simulink model "GRPsimWorkingPID"  (R2024b)
settings: Solver=FixedStepAuto  StartTime=0.0  StopTime=15  FixedStep=.0001  RelTol=1e-3
libraries: matrix_library x2, slpidlib x2, simulink x1, shared6dof x1
settings Model: Creator=aniketray  LastModifiedBy=aniketray

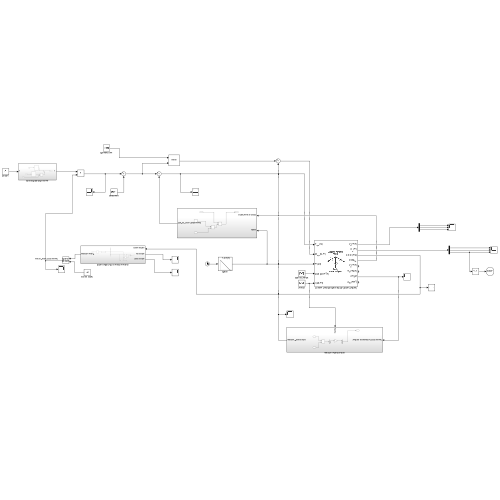
[thumbnail: Simulink's stored preview of the top-level diagram]
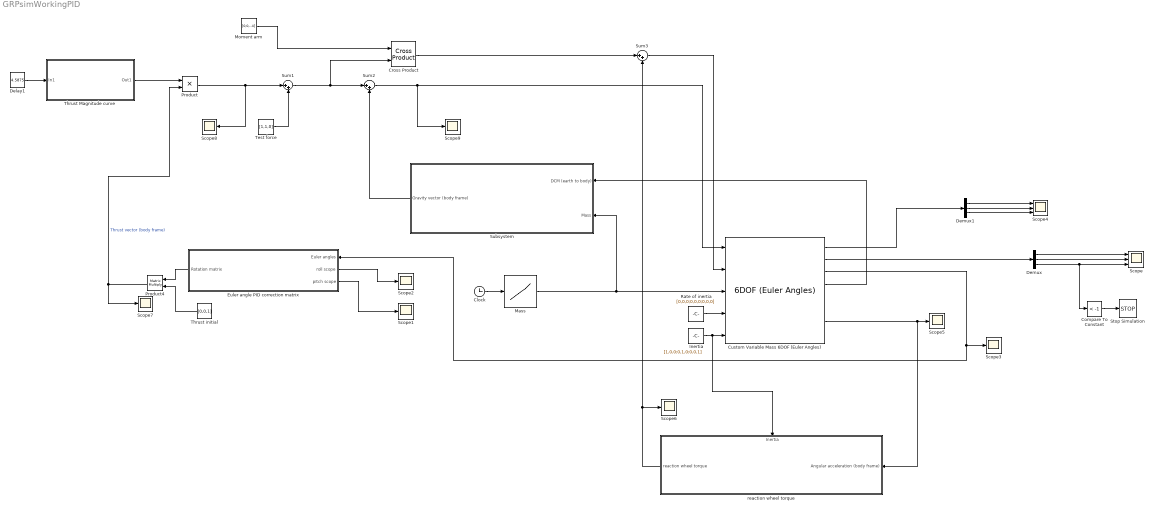
== system GRPsimWorkingPID ==
  Clock : Clock
  Compare To Constant : simulink/Logic and Bit Operations/Compare To Constant  relop=<  const=-1  OutDataTypeStr=boolean
  Cross Product : matrix_library/Cross Product
  Custom Variable Mass 6DOF (Euler Angles) : shared6dof/6DOF (Euler Angles)  units=Metric (MKS)  mtype=Custom Variable  rep=Euler Angles  xme_0=[0 0 0]  Vm_0=[0 0 0]  eul_0=[0,0,0]  pm_0=[0 0 0]  mass_0=1.0  mass_e=0.5  mass_f=2.0  inertia=eye(3)  inertia_e=eye(3)  inertia_f=2*eye(3)  k_quat=1.0  vre_flag=off  abi_flag=off  aMode=0  xme_statename=''  Vm_statename=''  eul_statename=''  quat_statename=''  pm_statename=''  mass_statename=''
      settings: LibrarySourceBlock=aerolib6dof2/Custom Variable Mass 6DOF (Euler Angles)
  Delay1 : Constant  Value=4.5875
  Demux : Demux  Outputs=3
  Demux1 : Demux  Outputs=3
  Euler angle PID correction matrix : Subsystem
      settings: PortSchema="{\"entries\":[{\"content\":{\"sides\":[{\"content\":{\"connectorIds\":[\"Out3\"]},\"type\":\"ConnectorPlacement.EquallySpacedRectSide\",\"uuid\":\"4ccd5e81-a240-4cab-acd1-338a2978d205\"},{\"content\":{\"connectorIds\":[\"In1\",\"Out1\",\"Out2\"],\"side\":\"RIGHT\"},\"type\":\"ConnectorPlacement.EquallySpacedRectSide\",\"uuid\":\"d7567d63-1202-4d9d-801d-ff17514df0c0\"},{\"content\":{\"side\":\"TOP\"},\"type\":\"ConnectorPlacement.EquallySpacedRectSide\",\"uuid\":\"5df3b33a-8f82-4d1a-a425-55f6edba809c\"}]},\"type\":\"ConnectorPlacement.EquallySpacedConnector\",\"uuid\":\"f1e1a38e-7b59-4704-87fe-778c34e8f949\"}],\"packageUris\":[\"http://schema.mathworks.com/mf0/Connector/R2020b\"],\"version\":\"1.0\"}"
  Inertia : Constant  Value=[1,0,0;0,1,0;0,0,1]
  Mass : Lookup_n-D  NumberOfTableDimensions=1  BreakpointsForDimension1=[0,3.45, 4]  Table=[1.2+0.06,1.2, 1.2]  InternalRulePriority=Speed  RndMeth=Simplest
  Moment arm : Constant  Value=[0,0,-.4]
  Product : Product
  Product4 : Product  Multiplication=Matrix(*)
  Rate of inertia : Constant  Value=[0,0,0;0,0,0;0,0,0]
  Scope : Scope  NumInputPorts=3
  Scope{1..3,5..9} (8 alike) : Scope
  Scope4 : Scope  NumInputPorts=3
  Stop Simulation : Stop
  Subsystem : Subsystem
  Sum1 : Sum  Inputs=|++
  Sum2 : Sum  Inputs=|++
  Sum3 : Sum  Inputs=|++
  Test force : Constant  Value=[1,1,0]
  Thrust Magnitude curve : Subsystem
  Thrust initial : Constant  Value=[0,0,1]
  reaction wheel torque : Subsystem
      settings: PortSchema="{\"entries\":[{\"content\":{\"sides\":[{\"content\":{\"connectorIds\":[\"In1\"]},\"type\":\"ConnectorPlacement.EquallySpacedRectSide\",\"uuid\":\"46941002-b8ec-4e8b-b9ab-4b9579ab10b5\"},{\"content\":{\"connectorIds\":[\"Out1\"],\"side\":\"RIGHT\"},\"type\":\"ConnectorPlacement.EquallySpacedRectSide\",\"uuid\":\"1b2f1bb1-3d36-42b5-8b8e-f1ef3188e1b6\"},{\"content\":{\"connectorIds\":[\"In2\"],\"side\":\"TOP\"},\"type\":\"ConnectorPlacement.EquallySpacedRectSide\",\"uuid\":\"06d0f9d8-e2f9-43b1-897a-1ea954ff583c\"}]},\"type\":\"ConnectorPlacement.EquallySpacedConnector\",\"uuid\":\"b4c30b9c-3a46-4044-8574-7f149b1eb989\"}],\"packageUris\":[\"http://schema.mathworks.com/mf0/Connector/R2020b\"],\"version\":\"1.0\"}"
  wires:
  Demux/2 -> Scope/2
  Demux/3 -> Scope/3, Compare To Constant/1
  Demux/1 -> Scope/1
  Compare To Constant/1 -> Stop Simulation/1
  Rate of inertia/1 -> Custom Variable Mass 6DOF (Euler Angles)/4
  Inertia/1 -> reaction wheel torque/2(Inertia), Custom Variable Mass 6DOF (Euler Angles)/5
  Custom Variable Mass 6DOF (Euler Angles)/2 -> Demux/1
  Clock/1 -> Mass/1
  Mass/1 -> Custom Variable Mass 6DOF (Euler Angles)/3, Subsystem/2(Mass)
  Product/1 -> Sum1/1, Scope8/1
  Sum2/1 -> Custom Variable Mass 6DOF (Euler Angles)/1, Scope9/1
  Demux1/1 -> Scope4/1
  Demux1/2 -> Scope4/2
  Demux1/3 -> Scope4/3
  Custom Variable Mass 6DOF (Euler Angles)/1 -> Demux1/1
  Moment arm/1 -> Cross Product/1
  Cross Product/1 -> Sum3/1
  Sum3/1 -> Custom Variable Mass 6DOF (Euler Angles)/2
  Custom Variable Mass 6DOF (Euler Angles)/3 -> Euler angle PID correction matrix/1(Euler angles), Scope3/1
  Thrust initial/1 -> Product4/2
  Product4/1 -> Product/2, Scope7/1  "Thrust vector (body frame)"
  Custom Variable Mass 6DOF (Euler Angles)/7 -> reaction wheel torque/1(Angular acceleration (body frame)), Scope5/1
  Delay1/1 -> Thrust Magnitude curve/1(In1)
  Thrust Magnitude curve/1(Out1) -> Product/1
  Euler angle PID correction matrix/3(Rotation matrix) -> Product4/1
  Euler angle PID correction matrix/1(roll scope) -> Scope2/1
  Euler angle PID correction matrix/2(pitch scope) -> Scope1/1
  Custom Variable Mass 6DOF (Euler Angles)/4 -> Subsystem/1(DCM (earth to body))
  Subsystem/1(Gravity vector (body frame)) -> Sum2/2
  Sum1/1 -> Cross Product/2, Sum2/1
  Test force/1 -> Sum1/2
  reaction wheel torque/1(reaction wheel torque) -> Scope6/1, Sum3/2

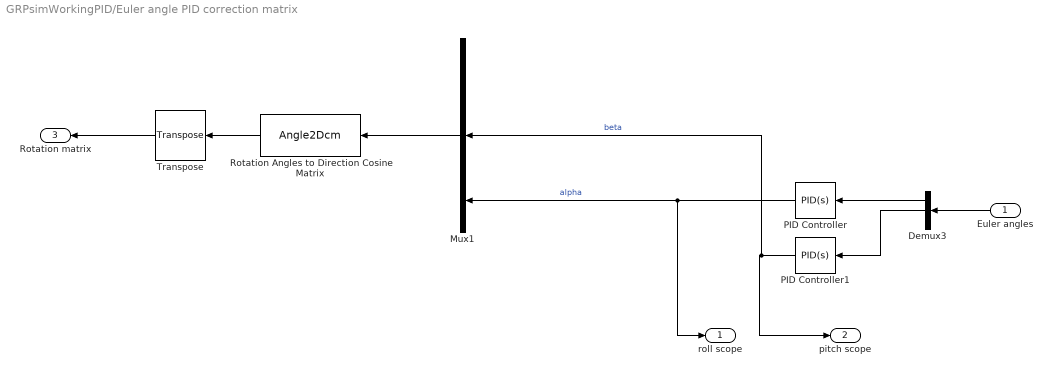
== system GRPsimWorkingPID/Euler angle PID correction matrix ==
  Euler angles : Inport
  Demux3 : Demux  Outputs=3
  Mux1 : Mux  Inputs=3
  PID Controller : slpidlib/PID Controller  Controller=PID  Form=Parallel  TimeDomain=Continuous-time  UseExternalTs=off  SampleTime=-1  IntegratorMethod=Forward Euler  FilterMethod=Forward Euler  ControllerParametersSource=internal  P=2.3  I=.2  UseKiTs=off  D=1.7  UseExternalDerivativeSource=off  N=100  UseFilter=on  TunerSelectOption=Transfer Function Based (PID Tuner App)  InitialConditionSource=internal  InitialConditionForIntegrator=0  InitialConditionForFilter=0  DifferentiatorICPrevScaledInput=0  ExternalReset=none  TrackingMode=off  Kt=1  LimitOutput=off  SatLimitsSource=internal  UpperSaturationLimit=inf  LowerSaturationLimit=-inf  LinearizeAsGain=on  AntiWindupMode=none  Kb=1  LimitIntegrator=off  UpperIntegratorSaturationLimit=inf  LowerIntegratorSaturationLimit=-inf  POutMin=[]  POutMax=[]  IOutMin=[]  IOutMax=[]  DOutMin=[]  DOutMax=[]  NOutMin=[]  NOutMax=[]  SumOutMin=[]  SumOutMax=[]  SaturationOutMin=[]  SaturationOutMax=[]  PParamMin=[]  PParamMax=[]  IParamMin=[]  IParamMax=[]  DParamMin=[]  DParamMax=[]  NParamMin=[]  NParamMax=[]  KbParamMin=[]  KbParamMax=[]  KtParamMin=[]  KtParamMax=[]  KbOutMin=[]  KbOutMax=[]  KtOutMin=[]  KtOutMax=[]  IntegratorOutMin=[]  IntegratorOutMax=[]  FilterOutMin=[]  FilterOutMax=[]  SumI1OutMin=[]  SumI1OutMax=[]  SumI2OutMin=[]  SumI2OutMax=[]  SumI3OutMin=[]  SumI3OutMax=[]  SumI4OutMin=[]  SumI4OutMax=[]  SumDOutMin=[]  SumDOutMax=[]  DifferentiatorOutMin=[]  DifferentiatorOutMax=[]  FilterDiffOutCoefMin=[]  FilterDiffOutCoefMax=[]  ReciprocalOutMin=[]  ReciprocalOutMax=[]  SumDenOutMin=[]  SumDenOutMax=[]  SumNumOutMin=[]  SumNumOutMax=[]  DivideOutMin=[]  DivideOutMax=[]  UdiffTsProdOutMin=[]  UdiffTsProdOutMax=[]  NTsProdOutMin=[]  NTsProdOutMax=[]  UintegralTsProdOutMin=[]  UintegralTsProdOutMax=[]  UngainTsProdOutMin=[]  UngainTsProdOutMax=[]  ClampingZeroOutDataTypeStr=Inherit: Inherit via back propagation  ClampingZeroOutMin=[]  ClampingZeroOutMax=[]  FilterDenConstantOutDataTypeStr=Inherit: Inherit via back propagation  FilterDenConstantOutMin=[]  FilterDenConstantOutMax=[]  PCopyOutDataTypeStr=Inherit: Inherit via back propagation  PCopyOutMin=[]  PCopyOutMax=[]  NCopyOutDataTypeStr=Inherit: Inherit via back propagation  NCopyOutMin=[]  NCopyOutMax=[]  IntegratorContinuousStateAttributes=''  IntegratorStateMustResolveToSignalObject=off  IntegratorRTWStateStorageClass=Auto  FilterContinuousStateAttributes=''  FilterStateMustResolveToSignalObject=off  FilterRTWStateStorageClass=Auto  ParallelPVariant=InternalParameters  IdealPVariant=Disabled  IVariant=InternalParameters  DVariant=InternalParameters  IntegratorVariant=Continuous  SatVariant=Disabled  AWVariant=Passthrough  PCopyVariant=Disabled  TRVariant=Disabled  FdbkBlocksVariant=Forward  IdealPFdbkVariant=Disabled  SatFdbkVariant=Disabled  DerivativeFilterVariant=ContFilter  NVariant=InternalParameters  NCopyVariant=Disabled  FilterICVariant=InternalICsFilter  IntegratorICVariant=InternalICs  ExternalResetVariant=Disabled  TRSumVariant=Passthrough  SumFdbkVariant=Disabled  SumVariant=Sum_PID  TsampFilterVariant=InternalTs  TsampNgainVariant=Passthrough  TsampIntegralVariant=Disabled_SignalSpec  ExternalSaturationOutDataTypeStr=Inherit: Same as second input  DerivativeSourceVariant=ErrorSignal  PreIntVariant=InternalPreInt
  PID Controller1 : slpidlib/PID Controller  Controller=PID  Form=Parallel  TimeDomain=Continuous-time  UseExternalTs=off  SampleTime=-1  IntegratorMethod=Forward Euler  FilterMethod=Forward Euler  ControllerParametersSource=internal  P=2.3  I=.2  UseKiTs=off  D=1.7  UseExternalDerivativeSource=off  N=100  UseFilter=on  TunerSelectOption=Transfer Function Based (PID Tuner App)  InitialConditionSource=internal  InitialConditionForIntegrator=0  InitialConditionForFilter=0  DifferentiatorICPrevScaledInput=0  ExternalReset=none  TrackingMode=off  Kt=1  LimitOutput=off  SatLimitsSource=internal  UpperSaturationLimit=inf  LowerSaturationLimit=-inf  LinearizeAsGain=on  AntiWindupMode=none  Kb=1  LimitIntegrator=off  UpperIntegratorSaturationLimit=inf  LowerIntegratorSaturationLimit=-inf  POutMin=[]  POutMax=[]  IOutMin=[]  IOutMax=[]  DOutMin=[]  DOutMax=[]  NOutMin=[]  NOutMax=[]  SumOutMin=[]  SumOutMax=[]  SaturationOutMin=[]  SaturationOutMax=[]  PParamMin=[]  PParamMax=[]  IParamMin=[]  IParamMax=[]  DParamMin=[]  DParamMax=[]  NParamMin=[]  NParamMax=[]  KbParamMin=[]  KbParamMax=[]  KtParamMin=[]  KtParamMax=[]  KbOutMin=[]  KbOutMax=[]  KtOutMin=[]  KtOutMax=[]  IntegratorOutMin=[]  IntegratorOutMax=[]  FilterOutMin=[]  FilterOutMax=[]  SumI1OutMin=[]  SumI1OutMax=[]  SumI2OutMin=[]  SumI2OutMax=[]  SumI3OutMin=[]  SumI3OutMax=[]  SumI4OutMin=[]  SumI4OutMax=[]  SumDOutMin=[]  SumDOutMax=[]  DifferentiatorOutMin=[]  DifferentiatorOutMax=[]  FilterDiffOutCoefMin=[]  FilterDiffOutCoefMax=[]  ReciprocalOutMin=[]  ReciprocalOutMax=[]  SumDenOutMin=[]  SumDenOutMax=[]  SumNumOutMin=[]  SumNumOutMax=[]  DivideOutMin=[]  DivideOutMax=[]  UdiffTsProdOutMin=[]  UdiffTsProdOutMax=[]  NTsProdOutMin=[]  NTsProdOutMax=[]  UintegralTsProdOutMin=[]  UintegralTsProdOutMax=[]  UngainTsProdOutMin=[]  UngainTsProdOutMax=[]  ClampingZeroOutDataTypeStr=Inherit: Inherit via back propagation  ClampingZeroOutMin=[]  ClampingZeroOutMax=[]  FilterDenConstantOutDataTypeStr=Inherit: Inherit via back propagation  FilterDenConstantOutMin=[]  FilterDenConstantOutMax=[]  PCopyOutDataTypeStr=Inherit: Inherit via back propagation  PCopyOutMin=[]  PCopyOutMax=[]  NCopyOutDataTypeStr=Inherit: Inherit via back propagation  NCopyOutMin=[]  NCopyOutMax=[]  IntegratorContinuousStateAttributes=''  IntegratorStateMustResolveToSignalObject=off  IntegratorRTWStateStorageClass=Auto  FilterContinuousStateAttributes=''  FilterStateMustResolveToSignalObject=off  FilterRTWStateStorageClass=Auto  ParallelPVariant=InternalParameters  IdealPVariant=Disabled  IVariant=InternalParameters  DVariant=InternalParameters  IntegratorVariant=Continuous  SatVariant=Disabled  AWVariant=Passthrough  PCopyVariant=Disabled  TRVariant=Disabled  FdbkBlocksVariant=Forward  IdealPFdbkVariant=Disabled  SatFdbkVariant=Disabled  DerivativeFilterVariant=ContFilter  NVariant=InternalParameters  NCopyVariant=Disabled  FilterICVariant=InternalICsFilter  IntegratorICVariant=InternalICs  ExternalResetVariant=Disabled  TRSumVariant=Passthrough  SumFdbkVariant=Disabled  SumVariant=Sum_PID  TsampFilterVariant=InternalTs  TsampNgainVariant=Passthrough  TsampIntegralVariant=Disabled_SignalSpec  ExternalSaturationOutDataTypeStr=Inherit: Same as second input  DerivativeSourceVariant=ErrorSignal  PreIntVariant=InternalPreInt
  Rotation Angles to Direction Cosine Matrix : Angle2Dcm
      settings: AttributesFormatString=Rotation Order: %<rotationOrder>
  Transpose : matrix_library/Transpose
  roll scope : Outport
  pitch scope : Outport  Port=2
  Rotation matrix : Outport  Port=3
  wires:
  Euler angles/1 -> Demux3/1
  Transpose/1 -> Rotation matrix/1
  Demux3/2 -> PID Controller1/1
  Mux1/1 -> Rotation Angles to Direction Cosine Matrix/1
  Demux3/1 -> PID Controller/1
  PID Controller/1 -> Mux1/3, roll scope/1  "alpha"
  PID Controller1/1 -> Mux1/2, pitch scope/1  "beta"
  Rotation Angles to Direction Cosine Matrix/1 -> Transpose/1

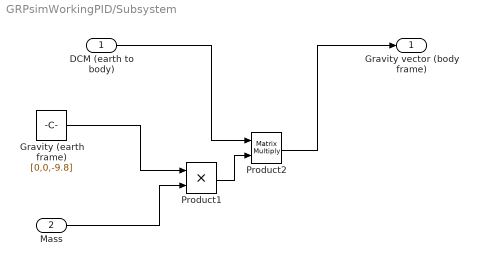
== system GRPsimWorkingPID/Subsystem ==
  DCM (earth to body) : Inport
  Mass : Inport  Port=2
  Gravity (earth frame) : Constant  Value=[0,0,-9.8]
  Product1 : Product
  Product2 : Product  Multiplication=Matrix(*)
  Gravity vector (body frame) : Outport
  wires:
  Product2/1 -> Gravity vector (body frame)/1
  Gravity (earth frame)/1 -> Product1/1
  Mass/1 -> Product1/2
  DCM (earth to body)/1 -> Product2/1
  Product1/1 -> Product2/2

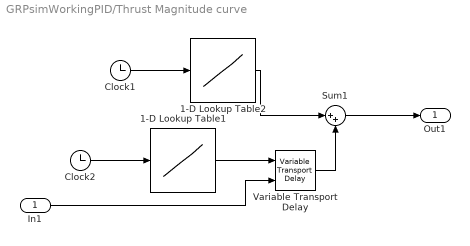
== system GRPsimWorkingPID/Thrust Magnitude curve ==
  In1 : Inport
  1-D Lookup Table1 : Lookup_n-D  NumberOfTableDimensions=1  BreakpointsForDimension1=[-10;0;0.063;0.11799999999999999;0.158;0.22800000000000001;0.34000000000000002;0.38600000000000001;0.42499999999999999;0.48099999999999998;0.58299999999999996;0.88300000000000001;1.1910000000000001;1.3640000000000001;1.569;1.7270000000000001;2;2.3900000000000001;2.6800000000000002;2.96;3.25;3.3500000000000001;3.3900000000000001;3.3999999999999999;10]  Table=[0;0;2.1269999999999998;4.407;8.359;13.68;20.82;26.75;25.379999999999999;22.190000000000001;17.93;16.109999999999999;14.59;15.35;15.65;14.74;14.279999999999999;13.68;13.08;13.07;13.050000000000001;13;7.2999999999999998;0;0]  InternalRulePriority=Speed  RndMeth=Simplest
  1-D Lookup Table2 : Lookup_n-D  NumberOfTableDimensions=1  BreakpointsForDimension1=[0;0.063;0.11799999999999999;0.158;0.22800000000000001;0.34000000000000002;0.38600000000000001;0.42499999999999999;0.48099999999999998;0.58299999999999996;0.88300000000000001;1.1910000000000001;1.3640000000000001;1.569;1.7270000000000001;2;2.3900000000000001;2.6800000000000002;2.96;3.25;3.3500000000000001;3.3900000000000001;3.3999999999999999;10]  Table=[0;2.1269999999999998;4.407;8.359;13.68;20.82;26.75;25.379999999999999;22.190000000000001;17.93;16.109999999999999;14.59;15.35;15.65;14.74;14.279999999999999;13.68;13.08;13.07;13.050000000000001;13;7.2999999999999998;0;0]  InternalRulePriority=Speed  RndMeth=Simplest
  Clock1 : Clock
  Clock2 : Clock
  Sum1 : Sum  Inputs=|++
  Variable Transport Delay : VariableTransportDelay  VariableDelayType=Variable transport delay  MaximumDelay=6  TransDelayFeedthrough=on
  Out1 : Outport
  wires:
  In1/1 -> Variable Transport Delay/2
  1-D Lookup Table2/1 -> Sum1/1
  Clock1/1 -> 1-D Lookup Table2/1
  Variable Transport Delay/1 -> Sum1/2
  1-D Lookup Table1/1 -> Variable Transport Delay/1
  Sum1/1 -> Out1/1
  Clock2/1 -> 1-D Lookup Table1/1

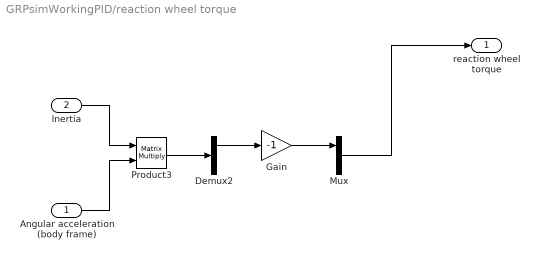
== system GRPsimWorkingPID/reaction wheel torque ==
  Angular acceleration (body frame) : Inport
  Inertia : Inport  Port=2
  Demux2 : Demux  Outputs=3
  Gain : Gain  Gain=-1
  Mux : Mux  Inputs=3
  Product3 : Product  Multiplication=Matrix(*)
  reaction wheel torque : Outport
  wires:
  Gain/1 -> Mux/1
  Inertia/1 -> Product3/1
  Product3/1 -> Demux2/1
  Angular acceleration (body frame)/1 -> Product3/2
  Demux2/1 -> Gain/1
  Mux/1 -> reaction wheel torque/1
